simulink model "MotorControlLibNEWFixedP_FULL"  (R2020b)
settings: Solver=FixedStepDiscrete  StartTime=0.0  StopTime=100  FixedStep=Ts  RelTol=1e-3
values from neighbouring files (symbols this model uses):
  Ki_Iab_EMFobs = 1600.0    [MotorControl.sldd]
  Kp_Iab_EMFobs = 0.255    [MotorControl.sldd]
  p = 8/2    (= 4)    [MotorControlLibData.m]    (also in local_pmsm_torque_control_data.m = 8)
  Ts = 250.0e-06    (= 0.00025)    [MotorControlLibData.m]    (also in local_pmsm_torque_control_data.m = 5e-06)
undefined symbols (not defined in the file or in its folder): BrkPoints, CuttOffFreq_c, d_q_Voltage_Limiter_sat_neg, d_q_Voltage_Limiter_sat_pos, DiscIntNeverNeededParam, Down, dSoll, EMFobsLdGain, EMFobsRS, Ki_dAxis, Ki_qAxis, Kp_dAxis, Kp_qAxis, MaxBckEMFVol_sat_neg, MaxBckEMFVol_sat_pos, NumBits1, NumBits2, qSoll, Slope1, Slope2, TqToIqConst, TsIntern, Up
libraries: simulink x12, pid_lib x4, eePwmGenerator x3, simulink_extras x2
(part 2 of 2)

== system MotorControlLibNEWFixedP_FULL/Position observer/Low pass filter1 ==
  note: d/dt(i)
  note: Integrator
  In1 : Inport
  Add2 : Sum  Inputs=+-
  Constant : Constant  Value=Value  OutDataTypeStr=uint16
  Delay : Delay  DelayLength=1  InitialCondition=0
  Gain : Gain  Gain=Gain  ParamDataTypeStr=fixdt(1,16,2^-16,0)  OutDataTypeStr=fixdt(1,16,2^-14,0)  SaturateOnIntegerOverflow=on
  Product1 : Product  OutDataTypeStr=fixdt(1,16,2^-6,0)
  Sum : Sum  Inputs=|++  OutDataTypeStr=Inherit: Same as first input
  Unit Delay : UnitDelay  SampleTime=-1  HasFrameUpgradeWarning=on
  Output : Outport
  wires:
  Unit Delay/1 -> Add2/2
  Sum/1 -> Product1/1, Delay/1
  Delay/1 -> Sum/2
  Gain/1 -> Sum/1
  Product1/1 -> Unit Delay/1, Output/1
  Add2/1 -> Gain/1
  In1/1 -> Add2/1
  Constant/1 -> Product1/2

== system MotorControlLibNEWFixedP_FULL/Position observer/Low pass filter2 ==
  note: Integrator
  note: d/dt(i)
  In1 : Inport
  Add2 : Sum  Inputs=+-
  Constant : Constant  Value=Value  OutDataTypeStr=uint16
  Delay : Delay  DelayLength=1  InitialCondition=0
  Gain : Gain  Gain=Gain  ParamDataTypeStr=fixdt(1,16,2^-16,0)  OutDataTypeStr=fixdt(1,16,2^-14,0)  SaturateOnIntegerOverflow=on
  Product1 : Product  OutDataTypeStr=fixdt(1,16,2^-6,0)
  Sum : Sum  Inputs=|++  OutDataTypeStr=Inherit: Same as first input
  Unit Delay : UnitDelay  SampleTime=-1  HasFrameUpgradeWarning=on
  Output : Outport
  wires:
  Constant/1 -> Product1/2
  In1/1 -> Add2/1
  Add2/1 -> Gain/1
  Product1/1 -> Output/1, Unit Delay/1
  Gain/1 -> Sum/1
  Delay/1 -> Sum/2
  Sum/1 -> Delay/1, Product1/1
  Unit Delay/1 -> Add2/2

== system MotorControlLibNEWFixedP_FULL/Position observer/Low pass filter3 ==
  note: d/dt(i)
  note: Integrator
  In1 : Inport
  Add2 : Sum  Inputs=+-
  Constant : Constant  Value=Value  OutDataTypeStr=uint16
  Delay : Delay  DelayLength=1  InitialCondition=0
  Gain : Gain  Gain=Gain  ParamDataTypeStr=fixdt(1,16,2^-16,0)  OutDataTypeStr=fixdt(1,16,2^-14,0)  SaturateOnIntegerOverflow=on
  Product1 : Product  OutDataTypeStr=fixdt(1,16,2^-6,0)
  Sum : Sum  Inputs=|++  OutDataTypeStr=Inherit: Same as first input
  Unit Delay : UnitDelay  SampleTime=-1  HasFrameUpgradeWarning=on
  Output : Outport
  wires:
  Unit Delay/1 -> Add2/2
  Sum/1 -> Product1/1, Delay/1
  Delay/1 -> Sum/2
  Gain/1 -> Sum/1
  Product1/1 -> Unit Delay/1, Output/1
  Add2/1 -> Gain/1
  In1/1 -> Add2/1
  Constant/1 -> Product1/2

== system MotorControlLibNEWFixedP_FULL/Start up/Logic after motor is stoped ==
  In1 : Inport
  Compare To Zero : simulink/Logic and Bit Operations/Compare To Zero  relop===  OutDataTypeStr=boolean
  Detect Decrease : simulink/Logic and Bit Operations/Detect Decrease  vinit=0  OutDataTypeStr=boolean
  Enabled Subsystem : Subsystem  TreatAsAtomicUnit=on
  Enabled Subsystem1 : Subsystem  TreatAsAtomicUnit=on
  S-R Flip-Flop : simulink_extras/Flip Flops/S-R Flip-Flop  initial_condition=0
  S-R Flip-Flop1 : simulink_extras/Flip Flops/S-R Flip-Flop  initial_condition=0
  Terminator : Terminator
  Terminator1 : Terminator
  Unit Delay : UnitDelay  SampleTime=-1  HasFrameUpgradeWarning=on
  Unit Delay1 : UnitDelay  SampleTime=-1  HasFrameUpgradeWarning=on
  Out1 : Outport
  wires:
  Enabled Subsystem/1(Out1) -> S-R Flip-Flop1/1
  In1/1 -> Enabled Subsystem/1(In1), Compare To Zero/1
  S-R Flip-Flop/2 -> Terminator/1
  Enabled Subsystem1/1(Output) -> Out1/1, Unit Delay1/1
  S-R Flip-Flop/1 -> Enabled Subsystem/Enable
  S-R Flip-Flop1/1 -> Enabled Subsystem1/Enable, Unit Delay/1
  Unit Delay/1 -> S-R Flip-Flop/2
  Compare To Zero/1 -> S-R Flip-Flop/1
  S-R Flip-Flop1/2 -> Terminator1/1
  Unit Delay1/1 -> Detect Decrease/1
  Detect Decrease/1 -> S-R Flip-Flop1/2

== system MotorControlLibNEWFixedP_FULL/Start up/Simulate start up Theta ==
  note: Overflow danger
  In1 : Inport
  Abs : Abs
  Constant : Constant  Value=2*pi  OutDataTypeStr=fixdt(1,16,2^-8,0)
  Discrete-Time Integrator : DiscreteIntegrator  ExternalReset=rising  SampleTime=-1  OutDataTypeStr=fixdt(1,16,2^-8,0)  ICPrevOutput=DiscIntNeverNeededParam  ICPrevScaledInput=DiscIntNeverNeededParam
  Relational Operator : RelationalOperator  OutDataTypeStr=boolean  RndMeth=Simplest
  Unit Delay : UnitDelay  SampleTime=-1  HasFrameUpgradeWarning=on
  Out1 : Outport
  wires:
  Constant/1 -> Relational Operator/2
  Relational Operator/1 -> Unit Delay/1
  Unit Delay/1 -> Discrete-Time Integrator/2
  In1/1 -> Discrete-Time Integrator/1
  Discrete-Time Integrator/1 -> Out1/1, Abs/1
  Abs/1 -> Relational Operator/1

== system MotorControlLibNEWFixedP_FULL/CosSin/Sine-Cosine Lookup/Interpolation ==
  In1 : Inport
  In2 : Inport  Port=2
  Demux : Demux
  Product : Product  RndMeth=Simplest  OutDataTypeStr=Inherit: Same as first input
  Product1 : Product  RndMeth=Simplest  OutDataTypeStr=Inherit: Same as first input
  Sum3 : Sum  Inputs=|+-  RndMeth=Simplest  OutDataTypeStr=Inherit: Same as first input
  Sum4 : Sum  Inputs=|++  RndMeth=Simplest  OutDataTypeStr=Inherit: Same as first input
  Sum5 : Sum  Inputs=|+-  RndMeth=Simplest  OutDataTypeStr=Inherit: Same as first input
  Sum6 : Sum  Inputs=|++  RndMeth=Simplest  OutDataTypeStr=Inherit: Same as first input
  Out1 : Outport
  Out2 : Outport  Port=2
  wires:
  Sum4/1 -> Out1/1
  Sum6/1 -> Out2/1
  Demux/1 -> Sum3/1
  Sum5/1 -> Product1/1
  Demux/2 -> Sum3/2, Sum4/2
  In2/1 -> Product/2, Product1/2
  Product/1 -> Sum4/1
  Demux/4 -> Sum6/2, Sum5/2
  Product1/1 -> Sum6/1
  In1/1 -> Demux/1
  Sum3/1 -> Product/1
  Demux/3 -> Sum5/1

== system MotorControlLibNEWFixedP_FULL/CosSin/Sine-Cosine Lookup/WrapUp ==
  In1 : Inport
  Compare To Zero : simulink/Logic and Bit Operations/Compare To Zero  relop=<  OutDataTypeStr=boolean
  Data Type Conversion : DataTypeConversion  OutDataTypeStr=uint16  ConvertRealWorld=Stored Integer (SI)  RndMeth=Simplest
  If : If
  If Action Subsystem : Subsystem  TreatAsAtomicUnit=on
  If Action Subsystem1 : Subsystem  TreatAsAtomicUnit=on
  Merge : Merge
  convert_pu : Gain  Gain=1/(dlgSett.UpperSatLimit)  RndMeth=Simplest  OutDataTypeStr=Inherit: Same as input
  Out1 : Outport
  wires:
  In1/1 -> convert_pu/1
  If/1 -> If Action Subsystem/Action
  If/2 -> If Action Subsystem1/Action
  convert_pu/1 -> Compare To Zero/1, If Action Subsystem/1(In1), If Action Subsystem1/1(In1)
  If Action Subsystem/1(Out1) -> Merge/1
  If Action Subsystem1/1(Out1) -> Merge/2
  Compare To Zero/1 -> Data Type Conversion/1
  Data Type Conversion/1 -> If/1
  Merge/1 -> Out1/1

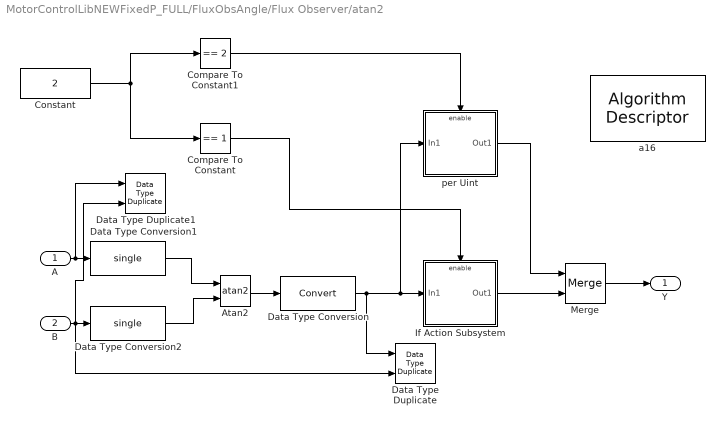
== system MotorControlLibNEWFixedP_FULL/FluxObsAngle/Flux Observer/atan2 ==
  A : Inport
  B : Inport  Port=2
  Atan2 : Trigonometry  Operator=atan2
  Compare To Constant : simulink/Logic and Bit Operations/Compare To Constant  relop===  const=1  OutDataTypeStr=boolean
  Compare To Constant1 : simulink/Logic and Bit Operations/Compare To Constant  relop===  const=2  OutDataTypeStr=boolean
  Constant : Constant  Value=2  OutDataTypeStr=uint16
  Data Type Duplicate : DataTypeDuplicate
  Data Type Duplicate1 : DataTypeDuplicate
  Data Type Conversion : DataTypeConversion
  Data Type Conversion1 : DataTypeConversion  OutDataTypeStr=single
  Data Type Conversion2 : DataTypeConversion  OutDataTypeStr=single
  If Action Subsystem : Subsystem  TreatAsAtomicUnit=on
  Merge : Merge
  a16 : AlgorithmDescriptor  AlgorithmName=trig_atan2  NumberOfInputs=2  InputBlockPath1=A  InputBlockPath2=B  ParameterBlockPath1=Constant  ParameterName1=Value  OutputBlockPath1=Y  OutputBlockPath2=Y2  NumberOfAlgorithmParameters=1  AlgorithmParameterName1=outputUnit  AlgorithmParameterValue1=PerUnit  AlgorithmParameterPrimary1=on
  per Uint : Subsystem  TreatAsAtomicUnit=on
  Y : Outport
  wires:
  Compare To Constant/1 -> If Action Subsystem/Enable
  Constant/1 -> Compare To Constant1/1, Compare To Constant/1
  Compare To Constant1/1 -> per Uint/Enable
  If Action Subsystem/1(Out1) -> Merge/2
  Atan2/1 -> Data Type Conversion/1
  per Uint/1(Out1) -> Merge/1
  Merge/1 -> Y/1
  A/1 -> Data Type Duplicate1/1, Data Type Conversion1/1
  B/1 -> Data Type Duplicate/2, Data Type Duplicate1/2, Data Type Conversion2/1
  Data Type Conversion1/1 -> Atan2/1
  Data Type Conversion2/1 -> Atan2/2
  Data Type Conversion/1 -> Data Type Duplicate/1, per Uint/1(In1), If Action Subsystem/1(In1)

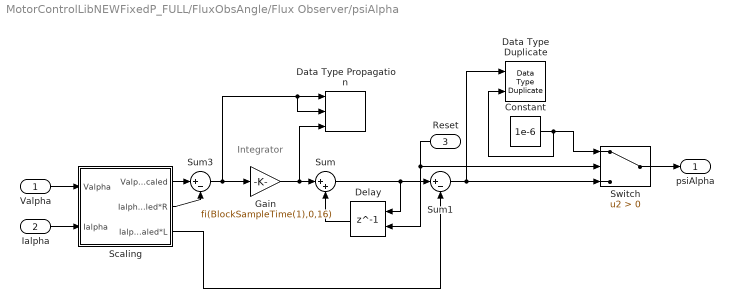
== system MotorControlLibNEWFixedP_FULL/FluxObsAngle/Flux Observer/psiAlpha ==
  note: Integrator
  Valpha : Inport
  Ialpha : Inport  Port=2
  Reset : Inport  Port=3
  Constant : Constant  Value=1e-6  OutDataTypeStr=Inherit: Inherit via back propagation
  Data Type Duplicate : DataTypeDuplicate
  Data Type Propagation : simulink/Signal Attributes/Data Type Propagation  PropDataType=fixdt(1, 16)  IfRefDouble=double  IfRefSingle=single  IsSigned=IsSigned1 or IsSigned2  NumBitsBase=max([NumBits1 NumBits2])  NumBitsMult=1  NumBitsAdd=0  NumBitsAllowFinal=1:128  PropScalingMode=Obtain via best precision  PropScaling=2^-10  ValuesUsedBestPrec=[4 -4]  SlopeBase=min([Slope1 Slope2])  SlopeMult=1  SlopeAdd=0  BiasBase=Bias1  BiasMult=1  BiasAdd=0
      settings: SourceProductBaseCode=SL
  Delay : Delay  DelayLength=1  ExternalReset=Level
      settings: InputPortMap=u0,r5
  Gain : Gain  Gain=fi(BlockSampleTime(1),0,16)  ParamDataTypeStr=Inherit: Inherit from 'Gain'  OutDataTypeStr=Inherit: Inherit via back propagation
  Scaling : Subsystem
  Sum : Sum  Inputs=|++  RndMeth=Simplest  OutDataTypeStr=Inherit: Same as first input
  Sum1 : Sum  Inputs=|+-  RndMeth=Simplest  OutDataTypeStr=Inherit: Same as first input
  Sum3 : Sum  Inputs=|+-  RndMeth=Simplest  OutDataTypeStr=Inherit: Same as first input
  Switch : Switch  Criteria=u2 > Threshold
  psiAlpha : Outport
  wires:
  Sum/1 -> Sum1/1, Delay/1
  Valpha/1 -> Scaling/1("Valpha ")
  Ialpha/1 -> Scaling/2(Ialpha)
  Scaling/1(ValphaScaled) -> Sum3/1
  Scaling/2(IalphaScaled*R) -> Sum3/2
  Delay/1 -> Sum/2
  Sum3/1 -> Data Type Propagation/2, Data Type Propagation/1, Gain/1
  Gain/1 -> Data Type Propagation/3, Sum/1
  Sum1/1 -> Switch/3, Data Type Duplicate/1
  Scaling/3(IalphaScaled*L) -> Sum1/2
  Reset/1 -> Delay/2, Switch/2
  Constant/1 -> Data Type Duplicate/2, Switch/1
  Switch/1 -> psiAlpha/1

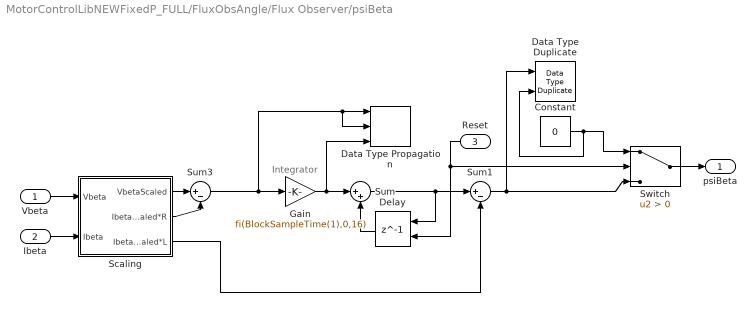
== system MotorControlLibNEWFixedP_FULL/FluxObsAngle/Flux Observer/psiBeta ==
  note: Integrator
  Vbeta : Inport
  Ibeta : Inport  Port=2
  Reset : Inport  Port=3
  Constant : Constant  Value=0  OutDataTypeStr=Inherit: Inherit via back propagation
  Data Type Duplicate : DataTypeDuplicate
  Data Type Propagation : simulink/Signal Attributes/Data Type Propagation  PropDataType=fixdt(1, 16)  IfRefDouble=double  IfRefSingle=single  IsSigned=IsSigned1 or IsSigned2  NumBitsBase=max([NumBits1 NumBits2])  NumBitsMult=1  NumBitsAdd=0  NumBitsAllowFinal=1:128  PropScalingMode=Obtain via best precision  PropScaling=2^-10  ValuesUsedBestPrec=[4 -4]  SlopeBase=min([Slope1 Slope2])  SlopeMult=1  SlopeAdd=0  BiasBase=Bias1  BiasMult=1  BiasAdd=0
      settings: SourceProductBaseCode=SL
  Delay : Delay  DelayLength=1  InitialCondition=0  ExternalReset=Level
      settings: InputPortMap=u0,r5
  Gain : Gain  Gain=fi(BlockSampleTime(1),0,16)  ParamDataTypeStr=Inherit: Inherit from 'Gain'  OutDataTypeStr=Inherit: Inherit via back propagation
  Scaling : Subsystem
  Sum : Sum  Inputs=|++  OutDataTypeStr=Inherit: Same as first input
  Sum1 : Sum  Inputs=|+-  RndMeth=Simplest  OutDataTypeStr=Inherit: Same as first input
  Sum3 : Sum  Inputs=|+-  RndMeth=Simplest  OutDataTypeStr=Inherit: Same as first input
  Switch : Switch  Criteria=u2 > Threshold
  psiBeta : Outport
  wires:
  Sum/1 -> Sum1/1, Delay/1
  Vbeta/1 -> Scaling/1(Vbeta)
  Ibeta/1 -> Scaling/2(Ibeta)
  Scaling/2(IbetaScaled*R) -> Sum3/2
  Scaling/1(VbetaScaled) -> Sum3/1
  Delay/1 -> Sum/2
  Sum3/1 -> Data Type Propagation/2, Data Type Propagation/1, Gain/1
  Gain/1 -> Data Type Propagation/3, Sum/1
  Reset/1 -> Delay/2, Switch/2
  Scaling/3(IbetaScaled*L) -> Sum1/2
  Sum1/1 -> Data Type Duplicate/1, Switch/3
  Switch/1 -> psiBeta/1
  Constant/1 -> Data Type Duplicate/2, Switch/1

== system MotorControlLibNEWFixedP_FULL/Position observer/EMF Observer Ia/DC Motor Model ==
  note: d/dt(i)
  note: Integrator
  Sig_Emfobs_PI_out : Inport
  In2 : Inport  Port=2
  In3 : Inport  Port=3
  Add5 : Sum  Inputs=-+--  OutDataTypeStr=Inherit: Same as first input
  Data Type Conversion : DataTypeConversion
  Delay : Delay  DelayLength=1  InitialCondition=0  StateName=UnitDelayIntegratorPosObs
  Gain : Gain  Gain=TsIntern  ParamDataTypeStr=Inherit: Inherit from 'Gain'  OutMin=-100  OutMax=+100  OutDataTypeStr=fixdt(1,16,2^-4,0)  SaturateOnIntegerOverflow=on
  Inductance : Gain  Gain=Ld  OutDataTypeStr=fixdt(1,16,2^9,0)
  Resistance : Gain  Gain=Rs  OutDataTypeStr=Inherit: Inherit via back propagation
  Sum : Sum  Inputs=|++  OutDataTypeStr=Inherit: Same as first input
  Unit Delay : UnitDelay  SampleTime=-1  HasFrameUpgradeWarning=on
  i_integrated_en8 : Outport
  wires:
  Unit Delay/1 -> Inductance/1
  Gain/1 -> Sum/1  "di_dt_times_Ts_En8"
  Sum/1 -> Delay/1, Data Type Conversion/1, Resistance/1  "i_integrated_en4"
  In2/1 -> Add5/2
  Resistance/1 -> Add5/1  "i_integrated_times_Rs_en8"
  Delay/1 -> Sum/2
  Sig_Emfobs_PI_out/1 -> Add5/3
  Add5/1 -> Unit Delay/1  "Va_all_16En4"
  Inductance/1 -> Gain/1  "di_dt_E9"
  Data Type Conversion/1 -> i_integrated_en8/1
  In3/1 -> Add5/4

== system MotorControlLibNEWFixedP_FULL/Position observer/EMF Observer Ia/PI Controller ==
  Sig_Emfobs_errorSum_m : Inport
  reset : Inport  Port=2
  Abs : Abs
  Add1 : Sum
  Anti-windup : Subsystem
  Constant : Constant  Commented=on  Value=Kp_Iab_EMFobs
  Constant2 : Constant  Commented=on  Value=Ki_Iab_EMFobs
  Data Type Conversion : DataTypeConversion  Commented=on
  Ki activation treashold : Constant  Value=0.23  OutDataTypeStr=fixdt(1,16,2^-8,0)
  Kp : Gain  Gain=Kp_Iab_EMFobs  OutDataTypeStr=Inherit: Same as input
  PID Controller : pid_lib/PID Controller  Commented=on  Controller=PI  Form=Parallel  TimeDomain=Discrete-time  UseExternalTs=off  SampleTime=-1  IntegratorMethod=Forward Euler  FilterMethod=Forward Euler  ControllerParametersSource=external  P=1  I=1  D=0  UseFilter=on  N=100  TunerSelectOption=Transfer Function Based (PID Tuner App)  ZeroCross=off  InitialConditionSource=internal  InitialConditionForIntegrator=0  InitialConditionForFilter=0  DifferentiatorICPrevScaledInput=0  ExternalReset=none  TrackingMode=off  Kt=1  LimitOutput=on  SatLimitsSource=internal  UpperSaturationLimit=MaxBckEMFVol_sat_pos  LowerSaturationLimit=MaxBckEMFVol_sat_neg  LinearizeAsGain=on  AntiWindupMode=clamping  Kb=1  POutMin=[]  POutMax=[]  IOutMin=[]  IOutMax=[]  DOutMin=[]  DOutMax=[]  NOutMin=[]  NOutMax=[]  SumOutMin=[]  SumOutMax=[]  SaturationOutMin=[]  SaturationOutMax=[]  PParamMin=[]  PParamMax=[]  IParamMin=[]  IParamMax=[]  DParamMin=[]  DParamMax=[]  NParamMin=[]  NParamMax=[]  KbParamMin=[]  KbParamMax=[]  KtParamMin=[]  KtParamMax=[]  KbOutMin=[]  KbOutMax=[]  KtOutMin=[]  KtOutMax=[]  IntegratorOutMin=[]  IntegratorOutMax=[]  FilterOutMin=[]  FilterOutMax=[]  SumI1OutMin=[]  SumI1OutMax=[]  SumI2OutMin=[]  SumI2OutMax=[]  SumI3OutMin=[]  SumI3OutMax=[]  SumI4OutMin=[]  SumI4OutMax=[]  SumDOutMin=[]  SumDOutMax=[]  DifferentiatorOutMin=[]  DifferentiatorOutMax=[]  FilterDiffOutCoefMin=[]  FilterDiffOutCoefMax=[]  ReciprocalOutMin=[]  ReciprocalOutMax=[]  SumDenOutMin=[]  SumDenOutMax=[]  SumNumOutMin=[]  SumNumOutMax=[]  DivideOutMin=[]  DivideOutMax=[]  UdiffTsProdOutMin=[]  UdiffTsProdOutMax=[]  NTsProdOutMin=[]  NTsProdOutMax=[]  UintegralTsProdOutMin=[]  UintegralTsProdOutMax=[]  UngainTsProdOutMin=[]  UngainTsProdOutMax=[]  IntegratorContinuousStateAttributes=''  IntegratorStateMustResolveToSignalObject=off  IntegratorRTWStateStorageClass=Auto  FilterContinuousStateAttributes=''  FilterStateMustResolveToSignalObject=off  FilterRTWStateStorageClass=Auto  ParallelPVariant=ExternalParameters  IdealPVariant=Disabled  IVariant=ExternalParameters  DVariant=Disabled  IntegratorVariant=Discrete  SatVariant=Enabled  AWVariant=DiscClampingParallel  PCopyVariant=Disabled  TRVariant=Disabled  FdbkBlocksVariant=Forward  IdealPFdbkVariant=Disabled  SatFdbkVariant=Disabled  DerivativeFilterVariant=Disabled  NVariant=Disabled  NCopyVariant=Disabled_SignalSpec  FilterICVariant=Disabled  IntegratorICVariant=InternalICs  ExternalResetVariant=Disabled  TRSumVariant=Passthrough  SumFdbkVariant=Disabled  SumVariant=Sum_PI  TsampFilterVariant=InternalTs  TsampNgainVariant=Passthrough  TsampIntegralVariant=Passthrough  ExternalSaturationOutDataTypeStr=Inherit: Same as second input
  Relational Operator : RelationalOperator  Operator=<=  OutDataTypeStr=boolean  RndMeth=Simplest
  Saturation : Saturate  UpperLimit=MaxBckEMFVol_sat_pos  LowerLimit=MaxBckEMFVol_sat_neg
  Sig_Emfobs_PI_out : Outport
  wires:
  PID Controller/1 -> Data Type Conversion/1
  Kp/1 -> Add1/1
  Anti-windup/1(Out1) -> Add1/2
  Ki activation treashold/1 -> Relational Operator/2
  Add1/1 -> Saturation/1
  Relational Operator/1 -> Anti-windup/Enable
  Constant/1 -> PID Controller/2
  Constant2/1 -> PID Controller/3
  Data Type Conversion/1 -> ?
  Sig_Emfobs_errorSum_m/1 -> PID Controller/1, Anti-windup/1(In1), Abs/1, Kp/1
  Saturation/1 -> Sig_Emfobs_PI_out/1  "Sig_Emfobs_PI_out"
  Abs/1 -> Relational Operator/1
  reset/1 -> Anti-windup/2(In2)

== system MotorControlLibNEWFixedP_FULL/Position observer/EMF Observer Ia1/DC Motor Model ==
  note: Integrator
  note: d/dt(i)
  note: i
  In1 : Inport
  In2 : Inport  Port=2
  Add5 : Sum  Inputs=-+-  OutDataTypeStr=Inherit: Same as first input
  Delay : Delay  DelayLength=1  InitialCondition=0
  Gain : Gain  Gain=TsIntern  ParamDataTypeStr=Inherit: Inherit from 'Gain'  OutDataTypeStr=Inherit: Inherit via back propagation
  Inductance : Gain  Gain=Ld  OutDataTypeStr=Inherit: Same as input
  Resistance : Gain  Gain=Rs  OutDataTypeStr=Inherit: Inherit via back propagation
  Sum : Sum  Inputs=|++  OutDataTypeStr=Inherit: Same as first input
  Unit Delay : UnitDelay  SampleTime=-1  HasFrameUpgradeWarning=on
  Out1 : Outport
  wires:
  Gain/1 -> Sum/1
  Delay/1 -> Sum/2
  Inductance/1 -> Gain/1
  Sum/1 -> Resistance/1, Out1/1, Delay/1
  Resistance/1 -> Add5/1
  Unit Delay/1 -> Inductance/1
  In1/1 -> Add5/3
  Add5/1 -> Unit Delay/1
  In2/1 -> Add5/2

== system MotorControlLibNEWFixedP_FULL/Position observer/EMF Observer Ia1/PI Controller ==
  In1 : Inport
  In2 : Inport  Port=2
  Add1 : Sum
  Add6 : Sum  Inputs=-+  InputSameDT=on
  Anti-windup : Subsystem
  Constant1 : Constant  Value=0.8  OutDataTypeStr=fixdt(1,32,2^-8,0)
  Kp : Gain  Gain=Kp_Iab_EMFobs  OutDataTypeStr=Inherit: Same as input
  Relational Operator : RelationalOperator  Operator=<=  OutDataTypeStr=boolean  RndMeth=Simplest
  Saturation : Saturate  UpperLimit=MaxBckEMFVol_sat_pos  LowerLimit=MaxBckEMFVol_sat_neg
  Out1 : Outport
  wires:
  In2/1 -> Add6/2
  Add6/1 -> Anti-windup/1(In1), Relational Operator/1, Kp/1
  Anti-windup/1(Out1) -> Add1/2
  Constant1/1 -> Relational Operator/2
  In1/1 -> Add6/1
  Relational Operator/1 -> Anti-windup/Enable
  Add1/1 -> Saturation/1
  Kp/1 -> Add1/1
  Saturation/1 -> Out1/1

== system MotorControlLibNEWFixedP_FULL/Position observer/EMF Observer Ia2/DC Motor Model ==
  note: Integrator
  note: d/dt(i)
  note: i
  Sig_Emfobs_PI_out : Inport
  In2 : Inport  Port=2
  Sig_Emfobs_PI_out1 : Inport  Port=3
  Add5 : Sum  Inputs=-+--  OutDataTypeStr=Inherit: Same as first input
  Delay : Delay  DelayLength=1  InitialCondition=0
  Gain : Gain  Gain=TsIntern  ParamDataTypeStr=Inherit: Inherit from 'Gain'  OutMin=-100  OutMax=+100  OutDataTypeStr=fixdt(1,16,2^-4,0)  SaturateOnIntegerOverflow=on
  Inductance : Gain  Gain=Ld  OutDataTypeStr=fixdt(1,16,2^9,0)
  Resistance : Gain  Gain=Rs  OutDataTypeStr=Inherit: Inherit via back propagation
  Sum : Sum  Inputs=|++  OutDataTypeStr=Inherit: Same as first input
  Unit Delay : UnitDelay  SampleTime=-1  HasFrameUpgradeWarning=on
  i_integrated_en8 : Outport
  wires:
  Sum/1 -> Resistance/1, i_integrated_en8/1, Delay/1
  Inductance/1 -> Gain/1
  Add5/1 -> Unit Delay/1
  Sig_Emfobs_PI_out/1 -> Add5/3
  Delay/1 -> Sum/2
  Resistance/1 -> Add5/1
  In2/1 -> Add5/2
  Gain/1 -> Sum/1
  Unit Delay/1 -> Inductance/1
  Sig_Emfobs_PI_out1/1 -> Add5/4

== system MotorControlLibNEWFixedP_FULL/Position observer/EMF Observer Ia2/PI Controller ==
  Sig_Emfobs_errorSum_m : Inport
  reset : Inport  Port=2
  Abs : Abs
  Add1 : Sum
  Anti-windup : Subsystem
  Constant : Constant  Commented=on  Value=Kp_Iab_EMFobs
  Constant1 : Constant  Value=0.23  OutDataTypeStr=fixdt(1,16,2^-8,0)
  Constant2 : Constant  Commented=on  Value=Ki_Iab_EMFobs
  Data Type Conversion : DataTypeConversion  Commented=on
  Kp : Gain  Gain=Kp_Iab_EMFobs  ParamDataTypeStr=Inherit: Inherit from 'Gain'  OutDataTypeStr=Inherit: Same as input
  PID Controller : pid_lib/PID Controller  Commented=on  Controller=PI  Form=Parallel  TimeDomain=Discrete-time  UseExternalTs=off  SampleTime=-1  IntegratorMethod=Forward Euler  FilterMethod=Forward Euler  ControllerParametersSource=external  P=1  I=1  D=0  UseFilter=on  N=100  TunerSelectOption=Transfer Function Based (PID Tuner App)  ZeroCross=off  InitialConditionSource=internal  InitialConditionForIntegrator=0  InitialConditionForFilter=0  DifferentiatorICPrevScaledInput=0  ExternalReset=none  TrackingMode=off  Kt=1  LimitOutput=on  SatLimitsSource=internal  UpperSaturationLimit=MaxBckEMFVol_sat_pos  LowerSaturationLimit=MaxBckEMFVol_sat_neg  LinearizeAsGain=on  AntiWindupMode=clamping  Kb=1  POutMin=[]  POutMax=[]  IOutMin=[]  IOutMax=[]  DOutMin=[]  DOutMax=[]  NOutMin=[]  NOutMax=[]  SumOutMin=[]  SumOutMax=[]  SaturationOutMin=[]  SaturationOutMax=[]  PParamMin=[]  PParamMax=[]  IParamMin=[]  IParamMax=[]  DParamMin=[]  DParamMax=[]  NParamMin=[]  NParamMax=[]  KbParamMin=[]  KbParamMax=[]  KtParamMin=[]  KtParamMax=[]  KbOutMin=[]  KbOutMax=[]  KtOutMin=[]  KtOutMax=[]  IntegratorOutMin=[]  IntegratorOutMax=[]  FilterOutMin=[]  FilterOutMax=[]  SumI1OutMin=[]  SumI1OutMax=[]  SumI2OutMin=[]  SumI2OutMax=[]  SumI3OutMin=[]  SumI3OutMax=[]  SumI4OutMin=[]  SumI4OutMax=[]  SumDOutMin=[]  SumDOutMax=[]  DifferentiatorOutMin=[]  DifferentiatorOutMax=[]  FilterDiffOutCoefMin=[]  FilterDiffOutCoefMax=[]  ReciprocalOutMin=[]  ReciprocalOutMax=[]  SumDenOutMin=[]  SumDenOutMax=[]  SumNumOutMin=[]  SumNumOutMax=[]  DivideOutMin=[]  DivideOutMax=[]  UdiffTsProdOutMin=[]  UdiffTsProdOutMax=[]  NTsProdOutMin=[]  NTsProdOutMax=[]  UintegralTsProdOutMin=[]  UintegralTsProdOutMax=[]  UngainTsProdOutMin=[]  UngainTsProdOutMax=[]  IntegratorContinuousStateAttributes=''  IntegratorStateMustResolveToSignalObject=off  IntegratorRTWStateStorageClass=Auto  FilterContinuousStateAttributes=''  FilterStateMustResolveToSignalObject=off  FilterRTWStateStorageClass=Auto  ParallelPVariant=ExternalParameters  IdealPVariant=Disabled  IVariant=ExternalParameters  DVariant=Disabled  IntegratorVariant=Discrete  SatVariant=Enabled  AWVariant=DiscClampingParallel  PCopyVariant=Disabled  TRVariant=Disabled  FdbkBlocksVariant=Forward  IdealPFdbkVariant=Disabled  SatFdbkVariant=Disabled  DerivativeFilterVariant=Disabled  NVariant=Disabled  NCopyVariant=Disabled_SignalSpec  FilterICVariant=Disabled  IntegratorICVariant=InternalICs  ExternalResetVariant=Disabled  TRSumVariant=Passthrough  SumFdbkVariant=Disabled  SumVariant=Sum_PI  TsampFilterVariant=InternalTs  TsampNgainVariant=Passthrough  TsampIntegralVariant=Passthrough  ExternalSaturationOutDataTypeStr=Inherit: Same as second input
  Relational Operator : RelationalOperator  Operator=<=  OutDataTypeStr=boolean  RndMeth=Simplest
  Saturation : Saturate  UpperLimit=MaxBckEMFVol_sat_pos  LowerLimit=MaxBckEMFVol_sat_neg
  Sig_Emfobs_PI_out : Outport
  wires:
  Saturation/1 -> Sig_Emfobs_PI_out/1
  Sig_Emfobs_errorSum_m/1 -> Kp/1, Anti-windup/1(In1), Abs/1, PID Controller/1
  Data Type Conversion/1 -> ?
  Constant2/1 -> PID Controller/3
  Constant/1 -> PID Controller/2
  Relational Operator/1 -> Anti-windup/Enable
  Add1/1 -> Saturation/1
  Constant1/1 -> Relational Operator/2
  Anti-windup/1(Out1) -> Add1/2
  Kp/1 -> Add1/1
  PID Controller/1 -> Data Type Conversion/1
  Abs/1 -> Relational Operator/1
  reset/1 -> Anti-windup/2(In2)

== system MotorControlLibNEWFixedP_FULL/Start up/Logic after motor is stoped/Enabled Subsystem ==
  In1 : Inport
  Enable : EnablePort
  Detect Change : simulink/Logic and Bit Operations/Detect Change  vinit=0  OutDataTypeStr=boolean
  Out1 : Outport
  wires:
  Detect Change/1 -> Out1/1
  In1/1 -> Detect Change/1

== system MotorControlLibNEWFixedP_FULL/Start up/Logic after motor is stoped/Enabled Subsystem1 ==
  Enable : EnablePort
  Add : Sum  OutDataTypeStr=uint16
  Constant : Constant  OutDataTypeStr=uint8
  Constant1 : Constant  Value=10000  OutDataTypeStr=uint16
  Relational Operator : RelationalOperator  Operator=<=  OutDataTypeStr=boolean  RndMeth=Simplest
  Unit Delay1 : UnitDelay  SampleTime=-1  HasFrameUpgradeWarning=on
  Output : Outport
  wires:
  Add/1 -> Unit Delay1/1
  Unit Delay1/1 -> Relational Operator/1, Add/1
  Constant/1 -> Add/2
  Constant1/1 -> Relational Operator/2
  Relational Operator/1 -> Output/1

== system MotorControlLibNEWFixedP_FULL/CosSin/Sine-Cosine Lookup/WrapUp/If Action Subsystem ==
  In1 : Inport
  Action Port : ActionPort
  Convert_back : DataTypeConversion  RndMeth=Simplest
  Convert_uint16 : DataTypeConversion  OutDataTypeStr=int16
  Data Type Duplicate : DataTypeDuplicate
  Sum : Sum  Inputs=|+-  RndMeth=Simplest  OutDataTypeStr=Inherit: Same as first input
  Out1 : Outport
  wires:
  In1/1 -> Convert_uint16/1, Sum/1, Data Type Duplicate/1
  Convert_back/1 -> Data Type Duplicate/2, Sum/2
  Sum/1 -> Out1/1
  Convert_uint16/1 -> Convert_back/1

== system MotorControlLibNEWFixedP_FULL/CosSin/Sine-Cosine Lookup/WrapUp/If Action Subsystem1 ==
  In1 : Inport
  Action Port : ActionPort
  Convert_back : DataTypeConversion  RndMeth=Simplest
  Convert_uint16 : DataTypeConversion  OutDataTypeStr=int16  RndMeth=Simplest
  Data Type Duplicate : DataTypeDuplicate
  Sum : Sum  Inputs=|+-  RndMeth=Simplest  OutDataTypeStr=Inherit: Same as first input
  Out1 : Outport
  wires:
  Convert_uint16/1 -> Convert_back/1
  Convert_back/1 -> Data Type Duplicate/2, Sum/2
  In1/1 -> Convert_uint16/1, Sum/1, Data Type Duplicate/1
  Sum/1 -> Out1/1

== system MotorControlLibNEWFixedP_FULL/FluxObsAngle/Flux Observer/atan2/If Action Subsystem ==
  In1 : Inport
  Enable : EnablePort
  Out1 : Outport
  wires:
  In1/1 -> Out1/1

== system MotorControlLibNEWFixedP_FULL/FluxObsAngle/Flux Observer/atan2/per Uint ==
  In1 : Inport
  Enable : EnablePort
  Bias : Bias  Bias=1
  Gain : Gain  Gain=1/(2*pi)  OutDataTypeStr=Inherit: Same as input
  Switch : Switch
  Out1 : Outport
  wires:
  In1/1 -> Gain/1
  Gain/1 -> Switch/2, Switch/1, Bias/1
  Switch/1 -> Out1/1
  Bias/1 -> Switch/3

== system MotorControlLibNEWFixedP_FULL/FluxObsAngle/Flux Observer/psiAlpha/Scaling ==
  "Valpha " : Inport
  Ialpha : Inport  Port=2
  ScalingL : Gain  Gain=StatorDAxisInductance  OutDataTypeStr=Inherit: Same as input
  ScalingR : Gain  Gain=StatorResistance  OutDataTypeStr=Inherit: Same as input
  ValphaScaled : Outport
  IalphaScaled*R : Outport  Port=2
  IalphaScaled*L : Outport  Port=3
  wires:
  ScalingR/1 -> IalphaScaled*R/1
  "Valpha "/1 -> ValphaScaled/1
  ScalingL/1 -> IalphaScaled*L/1
  Ialpha/1 -> ScalingL/1, ScalingR/1

== system MotorControlLibNEWFixedP_FULL/FluxObsAngle/Flux Observer/psiBeta/Scaling ==
  Vbeta : Inport
  Ibeta : Inport  Port=2
  ScalingL : Gain  Gain=StatorDAxisInductance  OutDataTypeStr=Inherit: Same as input
  ScalingR : Gain  Gain=StatorResistance  OutDataTypeStr=Inherit: Same as input
  VbetaScaled : Outport
  IbetaScaled*R : Outport  Port=2
  IbetaScaled*L : Outport  Port=3
  wires:
  ScalingR/1 -> IbetaScaled*R/1
  Vbeta/1 -> VbetaScaled/1
  ScalingL/1 -> IbetaScaled*L/1
  Ibeta/1 -> ScalingL/1, ScalingR/1

== system MotorControlLibNEWFixedP_FULL/Position observer/EMF Observer Ia/PI Controller/Anti-windup ==
  note: d/dt(i)
  note: Integrator
  In1 : Inport
  In2 : Inport  Port=2
  Enable : EnablePort
  Delay1 : Delay  DelayLength=1  InitialCondition=0  ExternalReset=Level
      settings: InputPortMap=u0,r5
  Gain1 : Gain  Gain=250e-6  ParamDataTypeStr=fixdt(1,16,2^-16,0)  OutDataTypeStr=fixdt(1,16,2^-12,0)
  Ki : Gain  Gain=Ki_Iab_EMFobs  ParamDataTypeStr=Inherit: Inherit from 'Gain'  OutDataTypeStr=Inherit: Same as input
  Sum1 : Sum  Inputs=|++  OutDataTypeStr=fixdt(1,16,2^-8,0)
  Out1 : Outport
  wires:
  Sum1/1 -> Out1/1, Delay1/1
  Gain1/1 -> Sum1/1
  Delay1/1 -> Sum1/2
  In1/1 -> Ki/1
  Ki/1 -> Gain1/1
  In2/1 -> Delay1/2

== system MotorControlLibNEWFixedP_FULL/Position observer/EMF Observer Ia1/PI Controller/Anti-windup ==
  note: Integrator
  note: d/dt(i)
  In1 : Inport
  Enable : EnablePort
  Delay1 : Delay  DelayLength=1  InitialCondition=0
  Gain1 : Gain  Gain=TsIntern  ParamDataTypeStr=Inherit: Inherit from 'Gain'  OutDataTypeStr=Inherit: Inherit via back propagation
  Ki : Gain  Gain=Ki_Iab_EMFobs  OutDataTypeStr=Inherit: Same as input
  Sum1 : Sum  Inputs=|++  OutDataTypeStr=Inherit: Same as first input
  Out1 : Outport
  wires:
  Ki/1 -> Gain1/1
  In1/1 -> Ki/1
  Delay1/1 -> Sum1/2
  Gain1/1 -> Sum1/1
  Sum1/1 -> Delay1/1, Out1/1

== system MotorControlLibNEWFixedP_FULL/Position observer/EMF Observer Ia2/PI Controller/Anti-windup ==
  note: Integrator
  note: d/dt(i)
  In1 : Inport
  In2 : Inport  Port=2
  Enable : EnablePort
  Delay1 : Delay  DelayLength=1  InitialCondition=0  ExternalReset=Level
      settings: InputPortMap=u0,r5
  Gain1 : Gain  Gain=250e-6  ParamDataTypeStr=fixdt(1,16,2^-16,0)  OutDataTypeStr=fixdt(1,16,2^-12,0)
  Ki : Gain  Gain=Ki_Iab_EMFobs  ParamDataTypeStr=Inherit: Inherit from 'Gain'  OutDataTypeStr=Inherit: Same as input
      settings: AttributesFormatString=%<Gain>
  Sum1 : Sum  Inputs=|++  OutDataTypeStr=fixdt(1,16,2^-8,0)
  Out1 : Outport
  wires:
  Ki/1 -> Gain1/1
  In1/1 -> Ki/1
  Delay1/1 -> Sum1/2
  Gain1/1 -> Sum1/1
  Sum1/1 -> Delay1/1, Out1/1
  In2/1 -> Delay1/2

== stateflow chart MotorControlLibNEWFixedP_FULL/Commented/Task Scheduler ==
  (default) -> (junction 23) : CLK_50us
  (junction 23) -> (junction 17)
  (junction 17) -> (junction 22) [order 2]
  (junction 17) -> (junction 22) [order 1] : [cnt%%2==0]{Task_100us_1;}
  (junction 22) -> (junction 18) [order 2]
  (junction 22) -> (junction 18) [order 1] : [cnt%%2==0]{Task_100us_2;}
  (junction 18) -> (junction 21) [order 1] : [cnt%%20==0]{Task_1ms_1;}
  (junction 18) -> (junction 21) [order 2]
  (junction 21) -> (junction 34) [order 2]
  (junction 21) -> (junction 16) [order 1] : [1]{cnt++;}
  data: cnt local int32
  events: Task_100us_1 output FUNCTION_CALL_EVENT; Task_100us_2 output FUNCTION_CALL_EVENT; Task_1ms_1 output FUNCTION_CALL_EVENT; CLK_50us input FUNCTION_CALL_EVENT

== stateflow chart MotorControlLibNEWFixedP_FULL/PI_Controller/Chart1 ==
  (default) -> (junction 6) : /* P Value ++ */
  (junction 6) -> (junction 19) [order 1] : [P==0]{P=0.00;}
  (junction 6) -> (junction 17) [order 2]
  (junction 19) -> (junction 17)
  (junction 17) -> (junction 24) [order 2]
  (junction 17) -> (junction 8) [order 1] : {P+=0.1;}
  (junction 8) -> (junction 11) [order 2] : [P<=5]
  (junction 11) -> (junction 13)
  (junction 8) -> (junction 9) [order 1] : [P>5]{P=5;}
  (junction 9) -> (junction 13)
  data: P output double

== stateflow chart MotorControlLibNEWFixedP_FULL/PI_Controller/Chart ==
  (default) -> (junction 6) : /* P Value ++ */
  (junction 6) -> (junction 8) : {P+=0.001;}
  (junction 8) -> (junction 11) [order 2] : [P<=0]
  (junction 11) -> (junction 13)
  (junction 8) -> (junction 9) [order 1] : [P>0]{P=0.02;}
  (junction 9) -> (junction 13)
  data: P output double

== stateflow chart MotorControlLibNEWFixedP_FULL/PI_Controller/Chart2 ==
  (default) -> (junction 6) : /* P Value ++ */
  (junction 6) -> (junction 8) : {P+=1;}
  (junction 8) -> (junction 11) [order 2] : [P<=0]
  (junction 11) -> (junction 13)
  (junction 8) -> (junction 9) [order 1] : [P>0]{P=4;}
  (junction 9) -> (junction 13)
  data: P output double
